simulink model "MOT_CTRL_PTH_FUN_002_1"  (R2025a)
settings: Solver=VariableStepAuto  StartTime=0.0  StopTime=10.0  RelTol=1e-3
settings Model: DataDictionary=Hbridge.sldd  Creator=tecnicomcbti  LastModifiedBy=tecnicomcbti

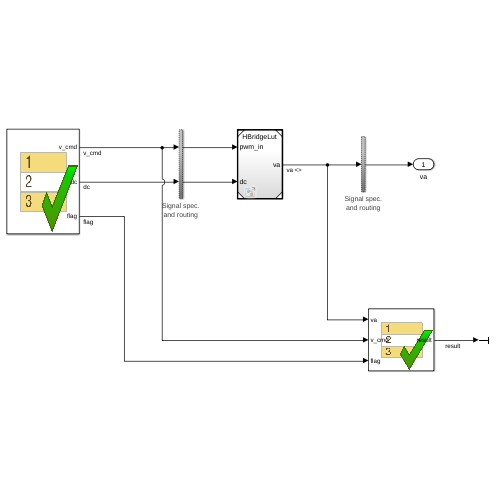
[thumbnail: Simulink's stored preview of the top-level diagram]
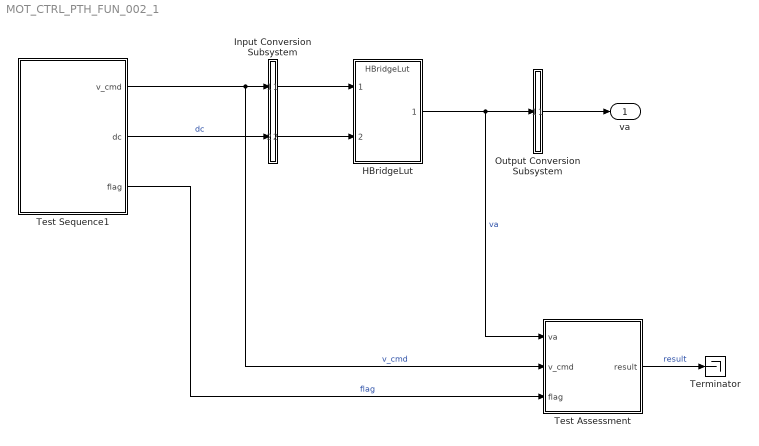
== system MOT_CTRL_PTH_FUN_002_1 ==
  HBridgeLut : ModelReference  ModelNameDialog=HBridgeLut  SimulationMode=Normal  ModelReferenceVersion=1.7
  Input Conversion Subsystem : Subsystem  Tag=__SLT_ICS__  Description=|
      | Signal spec.
      | and routing
      settings: AttributesFormatString=%<Description>
  Output Conversion Subsystem : Subsystem  Tag=__SLT_OCS__  Description=|
      | Signal spec.
      | and routing
      settings: AttributesFormatString=%<Description>
  Terminator : Terminator
  Test Assessment : Test Sequence  TreatAsAtomicUnit=on
  Test Sequence1 : Test Sequence  TreatAsAtomicUnit=on
  va : Outport
  wires:
  Output Conversion Subsystem/1(Outport_1) -> va/1
  Input Conversion Subsystem/1(Outport_1) -> HBridgeLut/1
  Input Conversion Subsystem/2(Outport_2) -> HBridgeLut/2
  HBridgeLut/1 -> Test Assessment/1(va), Output Conversion Subsystem/1(Inport_1)  "va"
  Test Assessment/1(result) -> Terminator/1  "result"
  Test Sequence1/1(v_cmd) -> Test Assessment/2(v_cmd), Input Conversion Subsystem/1(Inport_1)  "v_cmd"
  Test Sequence1/2(dc) -> Input Conversion Subsystem/2(Inport_2)  "dc"
  Test Sequence1/3(flag) -> Test Assessment/3(flag)  "flag"

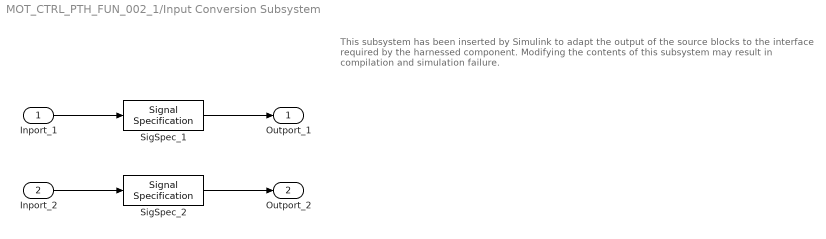
== system MOT_CTRL_PTH_FUN_002_1/Input Conversion Subsystem ==
  note: This subsystem has been inserted by Simulink to adapt the output of the source blocks to the interface required by the harnessed component.
      |  Modifying the contents of this subsystem may result in compilation and simulation failure.
  Inport_1 : Inport
  Inport_2 : Inport  Port=2
  SigSpec_1 : SignalSpecification  OutDataTypeStr=double  Dimensions=[1]  SampleTime=[0, 0]
  SigSpec_2 : SignalSpecification  OutDataTypeStr=double  Dimensions=[1]  SampleTime=[0, 0]
  Outport_1 : Outport
  Outport_2 : Outport  Port=2
  wires:
  SigSpec_1/1 -> Outport_1/1
  Inport_1/1 -> SigSpec_1/1
  SigSpec_2/1 -> Outport_2/1
  Inport_2/1 -> SigSpec_2/1

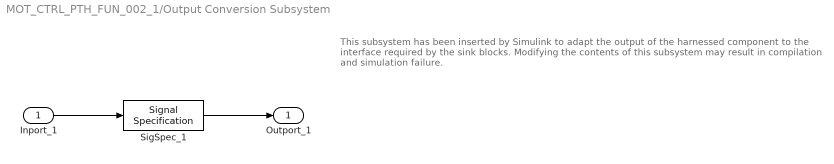
== system MOT_CTRL_PTH_FUN_002_1/Output Conversion Subsystem ==
  note: This subsystem has been inserted by Simulink to adapt the output of the harnessed component to the interface required by the sink blocks.
      |  Modifying the contents of this subsystem may result in compilation and simulation failure.
  Inport_1 : Inport
  SigSpec_1 : SignalSpecification  OutDataTypeStr=double  Dimensions=[1]
  Outport_1 : Outport
  wires:
  Inport_1/1 -> SigSpec_1/1
  SigSpec_1/1 -> Outport_1/1

== stateflow chart MOT_CTRL_PTH_FUN_002_1/Test Assessment ==
  state step_1
    state step_1_1
      if(va>(v_max*percent))
      result=true;
      else
      result=false;
      end
    state step_1_2
    (default) -> (junction 22)
    step_1 -> (junction 22)
    (junction 22) -> (junction 23) [order 1] : [(flag && (v_cmd>0))
        | ]
    (junction 23) -> step_1_1 [order 1] : [~in(step_1.step_1_1)]
    (junction 23) -> (junction 26) [order 2]
    (junction 31) -> (junction 32)
    (junction 32) -> step_1_2 [order 1] : [~in(step_1.step_1_2)]
    (junction 32) -> (junction 35) [order 2]
    (junction 22) -> (junction 31) [order 2]
  (default) -> step_1
  data: va input; v_cmd input; flag input boolean; result output boolean; percent constant double =0.9; v_max constant double =336

== stateflow chart MOT_CTRL_PTH_FUN_002_1/Test Sequence1 ==
  state Start
    v_cmd=0;
    dc=0;
    flag=false;
  state Set_positive
    v_cmd=5;
    dc=1;
    flag=true;
  (default) -> Start
  Start -> Set_positive : [
      | after(1,sec)
      | ]
  data: v_cmd output; dc output; flag output boolean
